simulink model "Problem_5"  (R2020b)
settings: Solver=VariableStepAuto  StartTime=0.0  StopTime=10.0  RelTol=1e-3
model workspace (MAT data in the model file):
  C = Simulink.Parameter
  C.Value = 1e-05
  C.DataType = 'auto'
  C.Dimensions = [1 1]
  R = Simulink.Parameter
  R.Value = 10
  R.DataType = 'auto'
  R.Dimensions = [1 1]
settings Model: Creator=Yeshwanth  LastModifiedBy=Yeshwanth

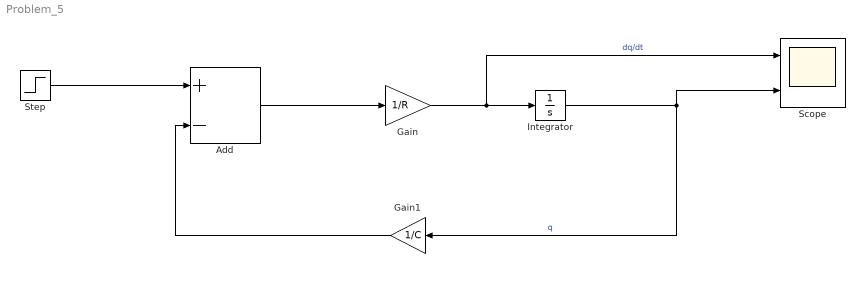
== system Problem_5 ==
  Add : Sum  Inputs=+-
  Gain : Gain  Gain=1/R
  Gain1 : Gain  Gain=1/C
  Integrator : Integrator
  Scope : Scope  NumInputPorts=2
  Step : Step  SampleTime=0
  wires:
  Gain1/1 -> Add/2
  Integrator/1 -> Scope/2, Gain1/1  "q"
  Add/1 -> Gain/1
  Gain/1 -> Scope/1, Integrator/1  "dq/dt"
  Step/1 -> Add/1
